simulink model "HLS_VMC_testing"  (R2025a)
settings: Solver=VariableStepAuto  StartTime=0.0  StopTime=0.0001  RelTol=1e-3
InitFcn:
  | fs = 500e6;
values from neighbouring files (symbols this model uses):
  N = length(X)    [outputPlots.m]
undefined symbols (not defined in the file or in its folder): A, es1, i, S, vsva2488, xcvr1602
libraries: hdlBasic x98, hlsBasic x64, aieUtilities x18, dspsrcs4 x15, dspxfrm3 x2, hdlDSPIP x2, hlsUtilities x1, vmcUtilities x1
(part 2 of 4)

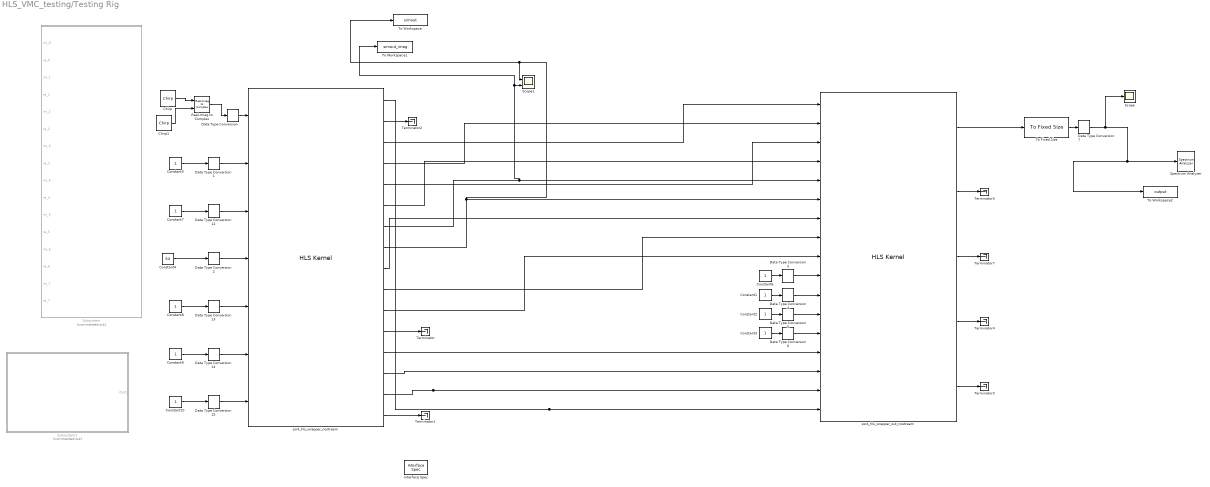
== system HLS_VMC_testing/Testing Rig ==
  Chirp : dspsrcs4/Chirp  sweep=Quadratic  mode=Unidirectional  f0=100e3  f1=100e6  t1=2048/fs  Tsweep=2048/fs  phase=0  Ts=1/fs  spf=1  datatype=double  OutputFrames=off
  Chirp1 : dspsrcs4/Chirp  sweep=Quadratic  mode=Unidirectional  f0=100e3  f1=100e6  t1=2048/fs  Tsweep=2048/fs  phase=pi  Ts=1/fs  spf=1  datatype=double  OutputFrames=off
  Constant{1..3,5..10} (9 alike) : Constant
  Constant4 : Constant  Value=54
  Data Type Conversion : hlsBasic/Data Type Conversion  OutDataType=data type expression  TypeExp='x_sfix64_En63'  Signedness=Signed  WordLength=16  FractionalLength=0  RoundingMode=Truncation to minus infinity  OverflowMode=Wrap around
  Data Type Conversion{1,12..15} (5 alike) : hlsBasic/Data Type Conversion  OutDataType=data type expression  TypeExp='x_ufix1'  Signedness=Signed  WordLength=16  FractionalLength=0  RoundingMode=Truncation to minus infinity  OverflowMode=Wrap around
  Data Type Conversion2 : hlsBasic/Data Type Conversion  OutDataType=data type expression  TypeExp='x_ufix18'  Signedness=Signed  WordLength=16  FractionalLength=0  RoundingMode=Truncation to minus infinity  OverflowMode=Wrap around
  Data Type Conversion{3..6} (4 alike) : hlsBasic/Data Type Conversion  OutDataType=data type expression  TypeExp='x_ufix12'  Signedness=Signed  WordLength=16  FractionalLength=0  RoundingMode=Truncation to minus infinity  OverflowMode=Wrap around
  Data Type Conversion7 : hlsBasic/Data Type Conversion  OutDataType=double  TypeExp=''  Signedness=Signed  WordLength=16  FractionalLength=0  RoundingMode=Truncation to minus infinity  OverflowMode=Wrap around
  Interface Spec : hlsUtilities/Interface Spec  Return=AXI4-Lite Slave@@  InportInterfaces={}  InportHandles={}  InportNames={}  OutportInterfaces={}  OutportHandles={}  OutportNames={}  Mode=AXI4-Lite Slave  InMode1=Default  InVFormat1=N/A  InVComponent1=N/A  InMode2=Default  InVFormat2=N/A  InVComponent2=N/A  InMode3=Default  InVFormat3=N/A  InVComponent3=N/A  InMode4=Default  InVFormat4=N/A  InVComponent4=N/A  InMode5=Default  InVFormat5=N/A  InVComponent5=N/A  InMode6=Default  InVFormat6=N/A  InVComponent6=N/A  InMode7=Default  InVFormat7=N/A  InVComponent7=N/A  InMode8=Default  InVFormat8=N/A  InVComponent8=N/A  OutMode1=Default  OutVFormat1=N/A  OutVComponent1=N/A  OutMode2=Default  OutVFormat2=N/A  OutVComponent2=N/A  OutMode3=Default  OutVFormat3=N/A  OutVComponent3=N/A  OutMode4=Default  OutVFormat4=N/A  OutVComponent4=N/A  OutMode5=Default  OutVFormat5=N/A  OutVComponent5=N/A  OutMode6=Default  OutVFormat6=N/A  OutVComponent6=N/A  OutMode7=Default  OutVFormat7=N/A  OutVComponent7=N/A  OutMode8=Default  OutVFormat8=N/A  OutVComponent8=N/A
  Real-Imag to Complex : hlsBasic/Real-Imag to Complex  Input=Real and imag  ConstantPart=0
  Scope : Scope
      settings: ActiveDisplayYMinimum=-1.249999998402562  ActiveDisplayYMaximum=1.2499999856230579  DataLoggingVariableName=ScopeData5
  Scope1 : Scope  NumInputPorts=2
      settings: ActiveDisplayYMinimum=-1.2499504089355469  ActiveDisplayYMaximum=1.2498588562011719  DataLoggingVariableName=ScopeData6
  Spectrum Analyzer : SpectrumAnalyzer  WindowPosition=[880.000000,470.000000,800.000000,500.000000,]  ScopeFrameLocation=window  WindowInvariantSamplesPerUpdate=on  Span=499999999.99999994  StartFrequency=-249999999.99999997  StopFrequency=249999999.99999997  YLimits=[-36.3231 18.9718]
  Subsystem : Subsystem  Commented=on
  Subsystem1 : Subsystem  Commented=on
  Terminator{,1..5,7} (7 alike) : Terminator
  To Fixed Size : aieUtilities/To Fixed Size  Mode=Stop simulation when input variable-size signal is not full  OutputSize=Inherit: Same as input  CopyMethod=Buffer samples to form output  HasStatusOutput=on
  To Workspace : ToWorkspace  VariableName=simout  SaveFormat=Structure With Time  SampleTime=1/fs
  To Workspace1 : ToWorkspace  VariableName=simout_imag  SaveFormat=Structure With Time  SampleTime=1/fs
  To Workspace2 : ToWorkspace  VariableName=output  SaveFormat=Structure With Time  SampleTime=-1
  ssr4_hls_wrapper_nostream : hlsBasic/HLS Kernel  PortNames={'return'; 'S_AXIS_din_tdata'; 'S_AXIS_din_tready_IN'; 'S_AXIS_din_tvalid_IN'; 'S_AXIS_din_tuser_IN'; 'S_AXIS_din_tlast_IN'; 'S_AXI_aresetn_IN'; 'S_AXI_enable_IN'; 'M_AXIS_dout_tready_OUT'; 'M_AXI_aresetn_OUT'; 'M_AXIS_din_tdata_sample_3_imag'; 'M_AXIS_din_tdata_sample_3_real'; 'M_AXIS_din_tdata_sample_2_imag'; 'M_AXIS_din_tdata_sample_2_real'; 'M_AXIS_din_tdata_sample_1_imag'; 'M_AXIS_din_tdata_sample_1_real'; 'M_AXIS_din_tdata_sample_0_imag'; 'M_AXIS_din_tdata_sample_0_real'; 'M_AXIS_din_tlast_OUT'; 'M_AXIS_din_tuser_scaling'; 'M_AXIS_din_tuser_direction'; 'M_AXIS_din_tuser_point_size'; 'M_AXIS_din_tvalid_OUT'; 'M_AXI_enable_OUT'}  PortSerializedTypes={'{Bv}'; '{R{Tstd::complex{1{t{Tap_fixed{5{t{}64}{t{}1}{t{}5}{t{}3}{t{}0}}}}}}}'; '{R{Tap_uint{1{t{}1}}}}'; '{R{Tap_uint{1{t{}1}}}}'; '{R{Tap_ufixed{5{t{}18}{t{}18}{t{}5}{t{}3}{t{}0}}}}'; '{R{Tap_uint{1{t{}1}}}}'; '{R{Tap_uint{1{t{}1}}}}'; '{R{Tap_uint{1{t{}1}}}}'; '{R{Tap_uint{1{t{}1}}}}'; '{R{Tap_uint{1{t{}1}}}}'; '{R{Tap_fixed{5{t{}16}{t{}1}{t{}0}{t{}3}{t{}0}}}}'; '{R{Tap_fixed{5{t{}16}{t{}1}{t{}0}{t{}3}{t{}0}}}}'; '{R{Tap_fixed{5{t{}16}{t{}1}{t{}0}{t{}3}{t{}0}}}}'; '{R{Tap_fixed{5{t{}16}{t{}1}{t{}0}{t{}3}{t{}0}}}}'; '{R{Tap_fixed{5{t{}16}{t{}1}{t{}0}{t{}3}{t{}0}}}}'; '{R{Tap_fixed{5{t{}16}{t{}1}{t{}0}{t{}3}{t{}0}}}}'; '{R{Tap_fixed{5{t{}16}{t{}1}{t{}0}{t{}3}{t{}0}}}}'; '{R{Tap_fixed{5{t{}16}{t{}1}{t{}0}{t{}3}{t{}0}}}}'; '{R{Tap_uint{1{t{}1}}}}'; '{R{Tap_ufixed{5{t{}13}{t{}1}{t{}5}{t{}3}{t{}0}}}}'; '{R{Tap_uint{1{t{}1}}}}'; '{R{Tap_uint{1{t{}4}}}}'; '{R{Tap_uint{1{t{}1}}}}'; '{R{Tap_uint{1{t{}1}}}}'}  FunctionTemplateSpecKind=none  FunctionTemplateParamNames={}  FunctionTemplateParamKinds={}  FunctionTemplateParamTypes={}  FunctionTemplateParamValues={}  PortSynchronicities={'sync'; 'sync'; 'sync'; 'sync'; 'sync'; 'sync'; 'sync'; 'sync'; 'sync'; 'sync'; 'sync'; 'sync'; 'sync'; 'sync'; 'sync'; 'sync'; 'sync'; 'sync'; 'sync'; 'sync'; 'sync'; 'sync'; 'sync'}  PortSignalSizes={0.000000000000000000e+00; 0.000000000000000000e+00; 0.000000000000000000e+00; 0.000000000000000000e+00; 0.000000000000000000e+00; 0.000000000000000000e+00; 0.000000000000000000e+00; 0.000000000000000000e+00; 0.000000000000000000e+00; 0.000000000000000000e+00; 0.000000000000000000e+00; 0.000000000000000000e+00; 0.000000000000000000e+00; 0.000000000000000000e+00; 0.000000000000000000e+00; 0.000000000000000000e+00; 0.000000000000000000e+00; 0.000000000000000000e+00; 0.000000000000000000e+00; 0.000000000000000000e+00; 0.000000000000000000e+00; 0.000000000000000000e+00; 0.000000000000000000e+00}  PortParameterValues={}  PortAttributesTable={ 'Input', 'S_AXIS_din_tdata', 'std::complex< ap_fixed< 64, 1, 5, 3, 0 > > &', 'sync', ''; 'Input', 'S_AXIS_din_tready_IN', 'ap_uint< 1 > &', 'sync', ''; 'Input', 'S_AXIS_din_tvalid_IN', 'ap_uint< 1 > &', 'sync', ''; 'Input', 'S_AXIS_din_tuser_IN', 'ap_ufixed< 18, 18, 5, 3, 0 > &', 'sync', ''; 'Input', 'S_AXIS_din_tlast_IN', 'ap_uint< 1 > &', 'sync', ''; 'Input', 'S_AXI_aresetn_IN', 'ap_uint< 1 > &', 'sync', ''; 'Input', 'S_AXI_enable_IN', 'ap_uint< 1 > &', 'sync', ''; 'Inout', 'M_AXIS_dout_tready_OUT', 'ap_uint< 1 > &', 'sync', ''; 'Inout', 'M_AXI_aresetn_OUT', 'ap_uint< 1 > &', 'sync', ''; 'Inout', 'M_AXIS_din_tdata_sample_3_imag', 'ap_fixed< 16, 1, 0, 3, 0 > &', 'sync', ''; 'Inout', 'M_AXIS_din_tdata_sample_3_real', 'ap_fixed< 16, 1, 0, 3, 0 > &', 'sync', ''; 'Inout', 'M_AXIS_din_tdata_sample_2_imag', 'ap_fixed< 16, 1, 0, 3, 0 > &', 'sync', ''; 'Inout', 'M_AXIS_din_tdata_sample_2_real', 'ap_fixed< 16, 1, 0, 3, 0 > &', 'sync', ''; 'Inout', 'M_AXIS_din_tdata_sample_1_imag', 'ap_fixed< 16, 1, 0, 3, 0 > &', 'sync', ''; 'Inout', 'M_AXIS_din_tdata_sample_1_real', 'ap_fixed< 16, 1, 0, 3, 0 > &', 'sync', ''; 'Inout', 'M_AXIS_din_tdata_sample_0_imag', 'ap_fixed< 16, 1, 0, 3, 0 > &', 'sync', ''; 'Inout', 'M_AXIS_din_tdata_sample_0_real', 'ap_fixed< 16, 1, 0, 3, 0 > &', 'sync', ''; 'Inout', 'M_AXIS_din_tlast_OUT', 'ap_uint< 1 > &', 'sync', ''; 'Inout', 'M_AXIS_din_tuser_scaling', 'ap_ufixed< 13, 1, 5, 3, 0 > &', 'sync', ''; 'Inout', 'M_AXIS_din_tuser_direction', 'ap_uint< 1 > &', 'sync', ''; 'Inout', 'M_AXIS_din_tuser_point_size', 'ap_uint< 4 > &', 'sync', ''; 'Inout', 'M_AXIS_din_tvalid_OUT', 'ap_uint< 1 > &', 'sync', ''; 'Inout', 'M_AXI_enable_OUT', 'ap_uint< 1 > &', 'sync', '' }  PortAttributesEnablement={'off', 'off', 'off', 'on', 'off';'off', 'off', 'off', 'on', 'off';'off', 'off', 'off', 'on', 'off';'off', 'off', 'off', 'on', 'off';'off', 'off', 'off', 'on', 'off';'off', 'off', 'off', 'on', 'off';'off', 'off', 'off', 'on', 'off';'off', 'off', 'off', 'on', 'off';'off', 'off', 'off', 'on', 'off';'off', 'off', 'off', 'on', 'off';'off', 'off', 'off', 'on', 'off';'off', 'off', 'off', 'on', 'off';'off', 'off', 'off', 'on', 'off';'off', 'off', 'off', 'on', 'off';'off', 'off', 'off', 'on', 'off';'off', 'off', 'off', 'on', 'off';'off', 'off', 'off', 'on', 'off';'off', 'off', 'off', 'on', 'off';'off', 'off', 'off', 'on', 'off';'off', 'off', 'off', 'on', 'off';'off', 'off', 'off', 'on', 'off';'off', 'off', 'off', 'on', 'off';'off', 'off', 'off', 'on', 'off'}  PortParametersTable={}  SampleTime=-1  PortDirectionTable={ 'S_AXIS_din_tdata', 'std::complex< ap_fixed< 64, 1, 5, 3, 0 > > &', 'Input', 'Port'; 'S_AXIS_din_tready_IN', 'ap_uint< 1 > &', 'Input', 'Port'; 'S_AXIS_din_tvalid_IN', 'ap_uint< 1 > &', 'Input', 'Port'; 'S_AXIS_din_tuser_IN', 'ap_ufixed< 18, 18, 5, 3, 0 > &', 'Input', 'Port'; 'S_AXIS_din_tlast_IN', 'ap_uint< 1 > &', 'Input', 'Port'; 'S_AXI_aresetn_IN', 'ap_uint< 1 > &', 'Input', 'Port'; 'S_AXI_enable_IN', 'ap_uint< 1 > &', 'Input', 'Port'; 'M_AXIS_dout_tready_OUT', 'ap_uint< 1 > &', 'Output', 'Port'; 'M_AXI_aresetn_OUT', 'ap_uint< 1 > &', 'Output', 'Port'; 'M_AXIS_din_tdata_sample_3_imag', 'ap_fixed< 16, 1, 0, 3, 0 > &', 'Output', 'Port'; 'M_AXIS_din_tdata_sample_3_real', 'ap_fixed< 16, 1, 0, 3, 0 > &', 'Output', 'Port'; 'M_AXIS_din_tdata_sample_2_imag', 'ap_fixed< 16, 1, 0, 3, 0 > &', 'Output', 'Port'; 'M_AXIS_din_tdata_sample_2_real', 'ap_fixed< 16, 1, 0, 3, 0 > &', 'Output', 'Port'; 'M_AXIS_din_tdata_sample_1_imag', 'ap_fixed< 16, 1, 0, 3, 0 > &', 'Output', 'Port'; 'M_AXIS_din_tdata_sample_1_real', 'ap_fixed< 16, 1, 0, 3, 0 > &', 'Output', 'Port'; 'M_AXIS_din_tdata_sample_0_imag', 'ap_fixed< 16, 1, 0, 3, 0 > &', 'Output', 'Port'; 'M_AXIS_din_tdata_sample_0_real', 'ap_fixed< 16, 1, 0, 3, 0 > &', 'Output', 'Port'; 'M_AXIS_din_tlast_OUT', 'ap_uint< 1 > &', 'Output', 'Port'; 'M_AXIS_din_tuser_scaling', 'ap_ufixed< 13, 1, 5, 3, 0 > &', 'Output', 'Port'; 'M_AXIS_din_tuser_direction', 'ap_uint< 1 > &', 'Output', 'Port'; 'M_AXIS_din_tuser_point_size', 'ap_uint< 4 > &', 'Output', 'Port'; 'M_AXIS_din_tvalid_OUT', 'ap_uint< 1 > &', 'Output', 'Port'; 'M_AXI_enable_OUT', 'ap_uint< 1 > &', 'Output', 'Port' }  FunctionTemplateParams={}  FunctionTemplateParamsEnables={}  FunctionTemplateParamsVisible=off  FunctionDeclTypeOptions=C[1 1]@t7@<empty>  PortDirectionTabVisible=on  ArgDirections={1.000000000000000000e+00; 1.000000000000000000e+00; 1.000000000000000000e+00; 1.000000000000000000e+00; 1.000000000000000000e+00; 1.000000000000000000e+00; 1.000000000000000000e+00; 2.000000000000000000e+00; 2.000000000000000000e+00; 2.000000000000000000e+00; 2.000000000000000000e+00; 2.000000000000000000e+00; 2.000000000000000000e+00; 2.000000000000000000e+00; 2.000000000000000000e+00; 2.000000000000000000e+00; 2.000000000000000000e+00; 2.000000000000000000e+00; 2.000000000000000000e+00; 2.000000000000000000e+00; 2.000000000000000000e+00; 2.000000000000000000e+00; 2.000000000000000000e+00}  ArgInterfaceTypes={1.000000000000000000e+00; 1.000000000000000000e+00; 1.000000000000000000e+00; 1.000000000000000000e+00; 1.000000000000000000e+00; 1.000000000000000000e+00; 1.000000000000000000e+00; 1.000000000000000000e+00; 1.000000000000000000e+00; 1.000000000000000000e+00; 1.000000000000000000e+00; 1.000000000000000000e+00; 1.000000000000000000e+00; 1.000000000000000000e+00; 1.000000000000000000e+00; 1.000000000000000000e+00; 1.000000000000000000e+00; 1.000000000000000000e+00; 1.000000000000000000e+00; 1.000000000000000000e+00; 1.000000000000000000e+00; 1.000000000000000000e+00; 1.000000000000000000e+00}  FunctionIndex=1  FormalArgDecls={'std::complex< ap_fixed< 64, 1, 5, 3, 0 > > & S_AXIS_din_tdata', 'ap_uint< 1 > & S_AXIS_din_tready_IN', 'ap_uint< 1 > & S_AXIS_din_tvalid_IN', 'ap_ufixed< 18, 18, 5, 3, 0 > & S_AXIS_din_tuser_IN', 'ap_uint< 1 > & S_AXIS_din_tlast_IN', 'ap_uint< 1 > & S_AXI_aresetn_IN', 'ap_uint< 1 > & S_AXI_enable_IN', 'ap_uint< 1 > & M_AXIS_dout_tready_OUT', 'ap_uint< 1 > & M_AXI_aresetn_OUT', 'ap_fixed< 16, 1, 0, 3, 0 > & M_AXIS_din_tdata_sample_3_imag', 'ap_fixed< 16, 1, 0, 3, 0 > & M_AXIS_din_tdata_sample_3_real', 'ap_fixed< 16, 1, 0, 3, 0 > & M_AXIS_din_tdata_sample_2_imag', 'ap_fixed< 16, 1, 0, 3, 0 > & M_AXIS_din_tdata_sample_2_real', 'ap_fixed< 16, 1, 0, 3, 0 > & M_AXIS_din_tdata_sample_1_imag', 'ap_fixed< 16, 1, 0, 3, 0 > & M_AXIS_din_tdata_sample_1_real', 'ap_fixed< 16, 1, 0, 3, 0 > & M_AXIS_din_tdata_sample_0_imag', 'ap_fixed< 16, 1, 0, 3, 0 > & M_AXIS_din_tdata_sample_0_real', 'ap_uint< 1 > & M_AXIS_din_tlast_OUT', 'ap_ufixed< 13, 1, 5, 3, 0 > & M_AXIS_din_tuser_scaling', 'ap_uint< 1 > & M_AXIS_din_tuser_direction', 'ap_uint< 4 > & M_AXIS_din_tuser_point_size', 'ap_uint< 1 > & M_AXIS_din_tvalid_OUT', 'ap_uint< 1 > & M_AXI_enable_OUT'}  SimLibPath=''  FunctionTabVisible=on  FunctionDescription=void ssr4_hls_wrapper_nostream(std::complex< ap_fixed< 64, 1, 5, 3, 0 > > & S_AXIS_din_tdata, ap_uint< 1 > & S_AXIS_din_tready_IN, ap_uint< 1 > & S_AXIS_din_tvalid_IN, ap_ufixed< 18, 18, 5, 3, 0 > & S_AXIS_din_tuser_IN, ap_uint< 1 > & S_AXIS_din_tlast_IN, ap_uint< 1 > & S_AXI_aresetn_IN, ap_uint< 1 > & S_AXI_enable_IN, ap_uint< 1 > & M_AXIS_dout_tready_OUT, ap_uint< 1 > & M_AXI_aresetn_OUT, ap_fixed< 16, 1, 0, 3, 0 > & M_AXIS_din_tdata_sample_3_imag, ap_fixed< 16, 1, 0, 3, 0 > & M_AXIS_din_tdata_sample_3_real, ap_fixed< 16, 1, 0, 3, 0 > & M_AXIS_din_tdata_sample_2_imag, ap_fixed< 16, 1, 0, 3, 0 > & M_AXIS_din_tdata_sample_2_real, ap_fixed< 16, 1, 0, 3, 0 > & M_AXIS_din_tdata_sample_1_imag, ap_fixed< 16, 1, 0, 3, 0 > & M_AXIS_din_tdata_sample_1_real, ap_fixed< 16, 1, 0, 3, 0 > & M_AXIS_din_tdata_sample_0_imag, ap_fixed< 16, 1, 0, 3, 0 > & M_AXIS_din_tdata_sample_0_real, ap_uint< 1 > & M_AXIS_din_tlast_OUT, ap_ufixed< 13, 1, 5, 3, 0 > & M_AXIS_din_tuser_scaling, ap_uint< 1 > & M_AXIS_din_tuser_direction, ap_uint< 4 > & M_AXIS_din_tuser_point_size, ap_uint< 1 > & M_AXIS_din_tvalid_OUT, ap_uint< 1 > & M_AXI_enable_OUT)  blockJsonConstraints=[]  deprecateConstraints=0  KernelHeaderFile=src/wrapperin.h  KernelFunction=ssr4_hls_wrapper_nostream  KernelFunctionSelect=<empty>  KernelSourceFile=src/wrapperin.cpp  KernelSearchPaths={}  PreProcOptions={}
  ssr4_hls_wrapper_out_nostream : hlsBasic/HLS Kernel  PortNames={'return'; 'S_AXIS_din_tdata_sample_3_imag'; 'S_AXIS_din_tdata_sample_3_real'; 'S_AXIS_din_tdata_sample_2_imag'; 'S_AXIS_din_tdata_sample_2_real'; 'S_AXIS_din_tdata_sample_1_imag'; 'S_AXIS_din_tdata_sample_1_real'; 'S_AXIS_din_tdata_sample_0_imag'; 'S_AXIS_din_tdata_sample_0_real'; 'S_AXIS_din_tlast_IN'; 'S_AXIS_din_tuser_index_3'; 'S_AXIS_din_tuser_index_2'; 'S_AXIS_din_tuser_index_1'; 'S_AXIS_din_tuser_index_0'; 'S_AXIS_din_tuser_direction'; 'S_AXIS_din_tuser_point_size'; 'S_AXIS_tvalid_IN'; 'S_AXIS_dout_tready_OUT'; 'M_AXIS_dout_tdata'; 'M_AXIS_dout_tlast_OUT'; 'M_AXIS_dout_tready_OUT'; 'M_AXIS_dout_tuser_OUT'; 'M_AXIS_dout_tvalid_OUT'}  PortSerializedTypes={'{Bv}'; '{R{Tap_fixed{5{t{}16}{t{}1}{t{}0}{t{}3}{t{}0}}}}'; '{R{Tap_fixed{5{t{}16}{t{}1}{t{}0}{t{}3}{t{}0}}}}'; '{R{Tap_fixed{5{t{}16}{t{}1}{t{}0}{t{}3}{t{}0}}}}'; '{R{Tap_fixed{5{t{}16}{t{}1}{t{}0}{t{}3}{t{}0}}}}'; '{R{Tap_fixed{5{t{}16}{t{}1}{t{}0}{t{}3}{t{}0}}}}'; '{R{Tap_fixed{5{t{}16}{t{}1}{t{}0}{t{}3}{t{}0}}}}'; '{R{Tap_fixed{5{t{}16}{t{}1}{t{}0}{t{}3}{t{}0}}}}'; '{R{Tap_fixed{5{t{}16}{t{}1}{t{}0}{t{}3}{t{}0}}}}'; '{R{Tap_uint{1{t{}1}}}}'; '{R{Tap_uint{1{t{}12}}}}'; '{R{Tap_uint{1{t{}12}}}}'; '{R{Tap_uint{1{t{}12}}}}'; '{R{Tap_uint{1{t{}12}}}}'; '{R{Tap_uint{1{t{}1}}}}'; '{R{Tap_uint{1{t{}4}}}}'; '{R{Tap_uint{1{t{}1}}}}'; '{R{Tap_uint{1{t{}1}}}}'; '{R{Tstd::complex{1{t{Tap_fixed{5{t{}64}{t{}1}{t{}0}{t{}3}{t{}0}}}}}}}'; '{R{Tap_uint{1{t{}1}}}}'; '{R{Tap_uint{1{t{}1}}}}'; '{R{Tap_uint{1{t{}53}}}}'; '{R{Tap_uint{1{t{}1}}}}'}  FunctionTemplateSpecKind=none  FunctionTemplateParamNames={}  FunctionTemplateParamKinds={}  FunctionTemplateParamTypes={}  FunctionTemplateParamValues={}  PortSynchronicities={'sync'; 'sync'; 'sync'; 'sync'; 'sync'; 'sync'; 'sync'; 'sync'; 'sync'; 'sync'; 'sync'; 'sync'; 'sync'; 'sync'; 'sync'; 'sync'; 'sync'; 'sync'; 'sync'; 'sync'; 'sync'; 'sync'}  PortSignalSizes={0.000000000000000000e+00; 0.000000000000000000e+00; 0.000000000000000000e+00; 0.000000000000000000e+00; 0.000000000000000000e+00; 0.000000000000000000e+00; 0.000000000000000000e+00; 0.000000000000000000e+00; 0.000000000000000000e+00; 0.000000000000000000e+00; 0.000000000000000000e+00; 0.000000000000000000e+00; 0.000000000000000000e+00; 0.000000000000000000e+00; 0.000000000000000000e+00; 0.000000000000000000e+00; 0.000000000000000000e+00; 0.000000000000000000e+00; 0.000000000000000000e+00; 0.000000000000000000e+00; 0.000000000000000000e+00; 0.000000000000000000e+00}  PortParameterValues={}  PortAttributesTable={ 'Input', 'S_AXIS_din_tdata_sample_3_imag', 'ap_fixed< 16, 1, 0, 3, 0 > &', 'sync', ''; 'Input', 'S_AXIS_din_tdata_sample_3_real', 'ap_fixed< 16, 1, 0, 3, 0 > &', 'sync', ''; 'Input', 'S_AXIS_din_tdata_sample_2_imag', 'ap_fixed< 16, 1, 0, 3, 0 > &', 'sync', ''; 'Input', 'S_AXIS_din_tdata_sample_2_real', 'ap_fixed< 16, 1, 0, 3, 0 > &', 'sync', ''; 'Input', 'S_AXIS_din_tdata_sample_1_imag', 'ap_fixed< 16, 1, 0, 3, 0 > &', 'sync', ''; 'Input', 'S_AXIS_din_tdata_sample_1_real', 'ap_fixed< 16, 1, 0, 3, 0 > &', 'sync', ''; 'Input', 'S_AXIS_din_tdata_sample_0_imag', 'ap_fixed< 16, 1, 0, 3, 0 > &', 'sync', ''; 'Input', 'S_AXIS_din_tdata_sample_0_real', 'ap_fixed< 16, 1, 0, 3, 0 > &', 'sync', ''; 'Input', 'S_AXIS_din_tlast_IN', 'ap_uint< 1 > &', 'sync', ''; 'Input', 'S_AXIS_din_tuser_index_3', 'ap_uint< 12 > &', 'sync', ''; 'Input', 'S_AXIS_din_tuser_index_2', 'ap_uint< 12 > &', 'sync', ''; 'Input', 'S_AXIS_din_tuser_index_1', 'ap_uint< 12 > &', 'sync', ''; 'Input', 'S_AXIS_din_tuser_index_0', 'ap_uint< 12 > &', 'sync', ''; 'Input', 'S_AXIS_din_tuser_direction', 'ap_uint< 1 > &', 'sync', ''; 'Input', 'S_AXIS_din_tuser_point_size', 'ap_uint< 4 > &', 'sync', ''; 'Input', 'S_AXIS_tvalid_IN', 'ap_uint< 1 > &', 'sync', ''; 'Input', 'S_AXIS_dout_tready_OUT', 'ap_uint< 1 > &', 'sync', ''; 'Inout', 'M_AXIS_dout_tdata', 'std::complex< ap_fixed< 64, 1, 0, 3, 0 > > &', 'sync', ''; 'Inout', 'M_AXIS_dout_tlast_OUT', 'ap_uint< 1 > &', 'sync', ''; 'Inout', 'M_AXIS_dout_tready_OUT', 'ap_uint< 1 > &', 'sync', ''; 'Inout', 'M_AXIS_dout_tuser_OUT', 'ap_uint< 53 > &', 'sync', ''; 'Inout', 'M_AXIS_dout_tvalid_OUT', 'ap_uint< 1 > &', 'sync', '' }  PortAttributesEnablement={'off', 'off', 'off', 'on', 'off';'off', 'off', 'off', 'on', 'off';'off', 'off', 'off', 'on', 'off';'off', 'off', 'off', 'on', 'off';'off', 'off', 'off', 'on', 'off';'off', 'off', 'off', 'on', 'off';'off', 'off', 'off', 'on', 'off';'off', 'off', 'off', 'on', 'off';'off', 'off', 'off', 'on', 'off';'off', 'off', 'off', 'on', 'off';'off', 'off', 'off', 'on', 'off';'off', 'off', 'off', 'on', 'off';'off', 'off', 'off', 'on', 'off';'off', 'off', 'off', 'on', 'off';'off', 'off', 'off', 'on', 'off';'off', 'off', 'off', 'on', 'off';'off', 'off', 'off', 'on', 'off';'off', 'off', 'off', 'on', 'off';'off', 'off', 'off', 'on', 'off';'off', 'off', 'off', 'on', 'off';'off', 'off', 'off', 'on', 'off';'off', 'off', 'off', 'on', 'off'}  PortParametersTable={}  SampleTime=-1  PortDirectionTable={ 'S_AXIS_din_tdata_sample_3_imag', 'ap_fixed< 16, 1, 0, 3, 0 > &', 'Input', 'Port'; 'S_AXIS_din_tdata_sample_3_real', 'ap_fixed< 16, 1, 0, 3, 0 > &', 'Input', 'Port'; 'S_AXIS_din_tdata_sample_2_imag', 'ap_fixed< 16, 1, 0, 3, 0 > &', 'Input', 'Port'; 'S_AXIS_din_tdata_sample_2_real', 'ap_fixed< 16, 1, 0, 3, 0 > &', 'Input', 'Port'; 'S_AXIS_din_tdata_sample_1_imag', 'ap_fixed< 16, 1, 0, 3, 0 > &', 'Input', 'Port'; 'S_AXIS_din_tdata_sample_1_real', 'ap_fixed< 16, 1, 0, 3, 0 > &', 'Input', 'Port'; 'S_AXIS_din_tdata_sample_0_imag', 'ap_fixed< 16, 1, 0, 3, 0 > &', 'Input', 'Port'; 'S_AXIS_din_tdata_sample_0_real', 'ap_fixed< 16, 1, 0, 3, 0 > &', 'Input', 'Port'; 'S_AXIS_din_tlast_IN', 'ap_uint< 1 > &', 'Input', 'Port'; 'S_AXIS_din_tuser_index_3', 'ap_uint< 12 > &', 'Input', 'Port'; 'S_AXIS_din_tuser_index_2', 'ap_uint< 12 > &', 'Input', 'Port'; 'S_AXIS_din_tuser_index_1', 'ap_uint< 12 > &', 'Input', 'Port'; 'S_AXIS_din_tuser_index_0', 'ap_uint< 12 > &', 'Input', 'Port'; 'S_AXIS_din_tuser_direction', 'ap_uint< 1 > &', 'Input', 'Port'; 'S_AXIS_din_tuser_point_size', 'ap_uint< 4 > &', 'Input', 'Port'; 'S_AXIS_tvalid_IN', 'ap_uint< 1 > &', 'Input', 'Port'; 'S_AXIS_dout_tready_OUT', 'ap_uint< 1 > &', 'Input', 'Port'; 'M_AXIS_dout_tdata', 'std::complex< ap_fixed< 64, 1, 0, 3, 0 > > &', 'Output', 'Port'; 'M_AXIS_dout_tlast_OUT', 'ap_uint< 1 > &', 'Output', 'Port'; 'M_AXIS_dout_tready_OUT', 'ap_uint< 1 > &', 'Output', 'Port'; 'M_AXIS_dout_tuser_OUT', 'ap_uint< 53 > &', 'Output', 'Port'; 'M_AXIS_dout_tvalid_OUT', 'ap_uint< 1 > &', 'Output', 'Port' }  FunctionTemplateParams={}  FunctionTemplateParamsEnables={}  FunctionTemplateParamsVisible=off  FunctionDeclTypeOptions=C[1 1]@t7@<empty>  PortDirectionTabVisible=on  ArgDirections={1.000000000000000000e+00; 1.000000000000000000e+00; 1.000000000000000000e+00; 1.000000000000000000e+00; 1.000000000000000000e+00; 1.000000000000000000e+00; 1.000000000000000000e+00; 1.000000000000000000e+00; 1.000000000000000000e+00; 1.000000000000000000e+00; 1.000000000000000000e+00; 1.000000000000000000e+00; 1.000000000000000000e+00; 1.000000000000000000e+00; 1.000000000000000000e+00; 1.000000000000000000e+00; 1.000000000000000000e+00; 2.000000000000000000e+00; 2.000000000000000000e+00; 2.000000000000000000e+00; 2.000000000000000000e+00; 2.000000000000000000e+00}  ArgInterfaceTypes={1.000000000000000000e+00; 1.000000000000000000e+00; 1.000000000000000000e+00; 1.000000000000000000e+00; 1.000000000000000000e+00; 1.000000000000000000e+00; 1.000000000000000000e+00; 1.000000000000000000e+00; 1.000000000000000000e+00; 1.000000000000000000e+00; 1.000000000000000000e+00; 1.000000000000000000e+00; 1.000000000000000000e+00; 1.000000000000000000e+00; 1.000000000000000000e+00; 1.000000000000000000e+00; 1.000000000000000000e+00; 1.000000000000000000e+00; 1.000000000000000000e+00; 1.000000000000000000e+00; 1.000000000000000000e+00; 1.000000000000000000e+00}  FunctionIndex=1  FormalArgDecls={'ap_fixed< 16, 1, 0, 3, 0 > & S_AXIS_din_tdata_sample_3_imag', 'ap_fixed< 16, 1, 0, 3, 0 > & S_AXIS_din_tdata_sample_3_real', 'ap_fixed< 16, 1, 0, 3, 0 > & S_AXIS_din_tdata_sample_2_imag', 'ap_fixed< 16, 1, 0, 3, 0 > & S_AXIS_din_tdata_sample_2_real', 'ap_fixed< 16, 1, 0, 3, 0 > & S_AXIS_din_tdata_sample_1_imag', 'ap_fixed< 16, 1, 0, 3, 0 > & S_AXIS_din_tdata_sample_1_real', 'ap_fixed< 16, 1, 0, 3, 0 > & S_AXIS_din_tdata_sample_0_imag', 'ap_fixed< 16, 1, 0, 3, 0 > & S_AXIS_din_tdata_sample_0_real', 'ap_uint< 1 > & S_AXIS_din_tlast_IN', 'ap_uint< 12 > & S_AXIS_din_tuser_index_3', 'ap_uint< 12 > & S_AXIS_din_tuser_index_2', 'ap_uint< 12 > & S_AXIS_din_tuser_index_1', 'ap_uint< 12 > & S_AXIS_din_tuser_index_0', 'ap_uint< 1 > & S_AXIS_din_tuser_direction', 'ap_uint< 4 > & S_AXIS_din_tuser_point_size', 'ap_uint< 1 > & S_AXIS_tvalid_IN', 'ap_uint< 1 > & S_AXIS_dout_tready_OUT', 'std::complex< ap_fixed< 64, 1, 0, 3, 0 > > & M_AXIS_dout_tdata', 'ap_uint< 1 > & M_AXIS_dout_tlast_OUT', 'ap_uint< 1 > & M_AXIS_dout_tready_OUT', 'ap_uint< 53 > & M_AXIS_dout_tuser_OUT', 'ap_uint< 1 > & M_AXIS_dout_tvalid_OUT'}  SimLibPath=''  FunctionTabVisible=on  FunctionDescription=void ssr4_hls_wrapper_out_nostream(ap_fixed< 16, 1, 0, 3, 0 > & S_AXIS_din_tdata_sample_3_imag, ap_fixed< 16, 1, 0, 3, 0 > & S_AXIS_din_tdata_sample_3_real, ap_fixed< 16, 1, 0, 3, 0 > & S_AXIS_din_tdata_sample_2_imag, ap_fixed< 16, 1, 0, 3, 0 > & S_AXIS_din_tdata_sample_2_real, ap_fixed< 16, 1, 0, 3, 0 > & S_AXIS_din_tdata_sample_1_imag, ap_fixed< 16, 1, 0, 3, 0 > & S_AXIS_din_tdata_sample_1_real, ap_fixed< 16, 1, 0, 3, 0 > & S_AXIS_din_tdata_sample_0_imag, ap_fixed< 16, 1, 0, 3, 0 > & S_AXIS_din_tdata_sample_0_real, ap_uint< 1 > & S_AXIS_din_tlast_IN, ap_uint< 12 > & S_AXIS_din_tuser_index_3, ap_uint< 12 > & S_AXIS_din_tuser_index_2, ap_uint< 12 > & S_AXIS_din_tuser_index_1, ap_uint< 12 > & S_AXIS_din_tuser_index_0, ap_uint< 1 > & S_AXIS_din_tuser_direction, ap_uint< 4 > & S_AXIS_din_tuser_point_size, ap_uint< 1 > & S_AXIS_tvalid_IN, ap_uint< 1 > & S_AXIS_dout_tready_OUT, std::complex< ap_fixed< 64, 1, 0, 3, 0 > > & M_AXIS_dout_tdata, ap_uint< 1 > & M_AXIS_dout_tlast_OUT, ap_uint< 1 > & M_AXIS_dout_tready_OUT, ap_uint< 53 > & M_AXIS_dout_tuser_OUT, ap_uint< 1 > & M_AXIS_dout_tvalid_OUT)  blockJsonConstraints=[]  deprecateConstraints=0  KernelHeaderFile=wrapper_out_src/wrapperout.h  KernelFunction=ssr4_hls_wrapper_out_nostream  KernelFunctionSelect=<empty>  KernelSourceFile=wrapper_out_src/wrapperout.cpp  KernelSearchPaths={}  PreProcOptions={}
  wires:
  ssr4_hls_wrapper_nostream/7 -> ssr4_hls_wrapper_out_nostream/5, To Workspace1/1, Scope1/2
  ssr4_hls_wrapper_nostream/11 -> ssr4_hls_wrapper_out_nostream/9
  ssr4_hls_wrapper_nostream/12 -> Terminator/1
  ssr4_hls_wrapper_nostream/13 -> ssr4_hls_wrapper_out_nostream/14
  ssr4_hls_wrapper_nostream/14 -> ssr4_hls_wrapper_out_nostream/15
  ssr4_hls_wrapper_nostream/15 -> ssr4_hls_wrapper_out_nostream/16
  ssr4_hls_wrapper_nostream/16 -> Terminator1/1
  ssr4_hls_wrapper_nostream/2 -> Terminator2/1
  Data Type Conversion2/1 -> ssr4_hls_wrapper_nostream/4
  Data Type Conversion1/1 -> ssr4_hls_wrapper_nostream/2
  Real-Imag to Complex/1 -> Data Type Conversion/1
  Constant4/1 -> Data Type Conversion2/1
  Constant5/1 -> Data Type Conversion1/1
  Data Type Conversion3/1 -> ssr4_hls_wrapper_out_nostream/10
  Constant6/1 -> Data Type Conversion3/1
  Data Type Conversion4/1 -> ssr4_hls_wrapper_out_nostream/11
  Constant1/1 -> Data Type Conversion4/1
  Data Type Conversion5/1 -> ssr4_hls_wrapper_out_nostream/12
  Constant2/1 -> Data Type Conversion5/1
  Data Type Conversion6/1 -> ssr4_hls_wrapper_out_nostream/13
  Constant3/1 -> Data Type Conversion6/1
  ssr4_hls_wrapper_nostream/8 -> ssr4_hls_wrapper_out_nostream/6, To Workspace/1, Scope1/1
  Chirp/1 -> Real-Imag to Complex/1
  Chirp1/1 -> Real-Imag to Complex/2
  Data Type Conversion/1 -> ssr4_hls_wrapper_nostream/1
  To Fixed Size/1 -> Data Type Conversion7/1
  Data Type Conversion7/1 -> Scope/1, To Workspace2/1, Spectrum Analyzer/1
  ssr4_hls_wrapper_nostream/1 -> ssr4_hls_wrapper_out_nostream/17
  Data Type Conversion12/1 -> ssr4_hls_wrapper_nostream/3
  Constant7/1 -> Data Type Conversion12/1
  Data Type Conversion13/1 -> ssr4_hls_wrapper_nostream/5
  Constant8/1 -> Data Type Conversion13/1
  Data Type Conversion14/1 -> ssr4_hls_wrapper_nostream/6
  Constant9/1 -> Data Type Conversion14/1
  Data Type Conversion15/1 -> ssr4_hls_wrapper_nostream/7
  Constant10/1 -> Data Type Conversion15/1
  ssr4_hls_wrapper_nostream/3 -> ssr4_hls_wrapper_out_nostream/1
  ssr4_hls_wrapper_nostream/4 -> ssr4_hls_wrapper_out_nostream/2
  ssr4_hls_wrapper_nostream/5 -> ssr4_hls_wrapper_out_nostream/3
  ssr4_hls_wrapper_nostream/6 -> ssr4_hls_wrapper_out_nostream/4
  ssr4_hls_wrapper_nostream/9 -> ssr4_hls_wrapper_out_nostream/7
  ssr4_hls_wrapper_nostream/10 -> ssr4_hls_wrapper_out_nostream/8
  ssr4_hls_wrapper_out_nostream/5 -> Terminator3/1
  ssr4_hls_wrapper_out_nostream/4 -> Terminator4/1
  ssr4_hls_wrapper_out_nostream/2 -> Terminator5/1
  ssr4_hls_wrapper_out_nostream/3 -> Terminator7/1
  ssr4_hls_wrapper_out_nostream/1 -> To Fixed Size/1

== system HLS_VMC_testing/Versal FFT HLS Wrapper ==
  S_AXIS_din_tdata : Inport
  " Scaling" : hdlBasic/Gateway In  gui_display_data_type=Fixed-point  arith_type=Unsigned  n_bits=13  bin_pt=13  preci_type=Single  exp_width=8  frac_width=24  rows=1  columns=1  quantization="Round  (unbiased: +/- Inf)"  overflow=Saturate  period=1/fs  UseAsADC=off  ADCChannel='1'  interface=None  automatic_assignment=on  address_offset=hex2dec('00')  intf_name=''  intf_description=''  default_value=0  timing_constraint=None  locs_specified=off  LOCs={}  io_standard={}  inherit_from_input=off  hdl_port=on  XmcBlockStatus=1  maskContainerNames=group4  block_type=gatewayin  block_config=sysgen:gateway_in_config  block_width_w=590  block_height_w=620  block_width=640  block_height=850
  Concat : hdlBasic/Concat  num_inputs=3  XmcBlockStatus=1  maskContainerNames=group1  block_type=concat  block_config=sysgen:Concat_config
  Direction : hdlBasic/Gateway In  gui_display_data_type=Boolean  arith_type=Boolean  n_bits=16  bin_pt=14  preci_type=Single  exp_width=8  frac_width=24  rows=1  columns=1  quantization="Round  (unbiased: +/- Inf)"  overflow=Saturate  period=1/fs  UseAsADC=off  ADCChannel='1'  interface=None  automatic_assignment=on  address_offset=hex2dec('00')  intf_name=''  intf_description=''  default_value=0  timing_constraint=None  locs_specified=off  LOCs={}  io_standard={}  inherit_from_input=off  hdl_port=on  XmcBlockStatus=1  maskContainerNames=group4  block_type=gatewayin  block_config=sysgen:gateway_in_config  block_width_w=590  block_height_w=620  block_width=640  block_height=850
  Display1 : Display
  Point Size : hdlBasic/Gateway In  gui_display_data_type=Fixed-point  arith_type=Unsigned  n_bits=4  bin_pt=0  preci_type=Single  exp_width=8  frac_width=24  rows=1  columns=1  quantization="Round  (unbiased: +/- Inf)"  overflow=Saturate  period=1/fs  UseAsADC=off  ADCChannel='1'  interface=None  automatic_assignment=on  address_offset=hex2dec('00')  intf_name=''  intf_description=''  default_value=0  timing_constraint=None  locs_specified=off  LOCs={}  io_standard={}  inherit_from_input=off  hdl_port=on  XmcBlockStatus=1  maskContainerNames=group4  block_type=gatewayin  block_config=sysgen:gateway_in_config  block_width_w=590  block_height_w=620  block_width=640  block_height=850
  Scope : Scope
      settings: ActiveDisplayYMinimum=-0.12499999999999997  ActiveDisplayYMaximum=1.125  DataLoggingVariableName=ScopeData3
  Shift : hdlBasic/Shift  shift_dir=Left  shift_bits=13  en=off  latency=0  precision=User Defined  arith_type=Unsigned  n_bits=13  bin_pt=0  quantization=Truncate  overflow=Wrap  XmcBlockStatus=1  maskContainerNames=group2  block_type=shift  block_config=sysgen:Shift_config
  TLAST_DELAY : DiscretePulseGenerator  Period=FFT_SIZE  PhaseDelay=FFT_SIZE - 1  SampleTime=1/fs
  TUSER_Direction : Constant  Value=tuser_dir  SampleTime=1/fs
  TUSER_PointSIze : Constant  Value=tuser_ps  SampleTime=1/fs
  TUSER_Scaling : Constant  Value=tuser  SampleTime=1/fs
  mask_level_wrapper : Subsystem
  M_AXIS_dout_tdata : Outport
  dout_tvalid : Outport  Port=2
  wires:
  mask_level_wrapper/1(M_AXIS_dout_tdata) -> M_AXIS_dout_tdata/1
  S_AXIS_din_tdata/1 -> mask_level_wrapper/1(S_AXIS_din_tdata)
  TUSER_Direction/1 -> Direction/1
  TUSER_PointSIze/1 -> Point Size/1
  TUSER_Scaling/1 -> " Scaling"/1
  Point Size/1 -> Concat/3
  Direction/1 -> Concat/2
  mask_level_wrapper/2(dout_tvalid) -> dout_tvalid/1
  Concat/1 -> mask_level_wrapper/2(S_AXIS_din_tuser)
  TLAST_DELAY/1 -> mask_level_wrapper/3(S_AXIS_din_tlast)
  " Scaling"/1 -> Shift/1
  Shift/1 -> Concat/1

== system HLS_VMC_testing/Versal FFT HLS Wrapper1 ==
  S_AXIS_din_tdata : Inport
  Constant : Constant  Value=tuser
  Constant1 : Constant  Value=tuser_dir
  Constant2 : Constant  Value=tuser_ps
  Data Type Conversion : hlsBasic/Data Type Conversion  OutDataType=double  TypeExp=''  Signedness=Signed  WordLength=16  FractionalLength=0  RoundingMode=Truncation to minus infinity  OverflowMode=Wrap around
  TLAST_DELAY : DiscretePulseGenerator  Period=FFT_SIZE  PhaseDelay=FFT_SIZE - 1  SampleTime=1/fs
  TUSER formatting : Subsystem
  mask_level_wrapper : Subsystem
  M_AXIS_dout_tdata : Outport
  M_AXIS_dout_tvalid : Outport  Port=2
  wires:
  mask_level_wrapper/1(M_AXIS_dout_tdata_) -> M_AXIS_dout_tdata/1
  S_AXIS_din_tdata/1 -> mask_level_wrapper/1(S_AXIS_din_tdata_)
  TLAST_DELAY/1 -> mask_level_wrapper/3(S_AXIS_din_tlast_)
  mask_level_wrapper/2(tvalid) -> M_AXIS_dout_tvalid/1
  TUSER formatting/1(S_AXIS_din_tuser_) -> Data Type Conversion/1
  Constant/1 -> TUSER formatting/1(In1)
  Constant1/1 -> TUSER formatting/2(In2)
  Constant2/1 -> TUSER formatting/3(In3)
  Data Type Conversion/1 -> mask_level_wrapper/2(S_AXIS_din_tuser_)

== system HLS_VMC_testing/Input Stimuli1/Pre Processing ==
  In1 : Inport
  Buffer2 : Buffer  N=1  OutputFrames=off
  Complex to Real-Imag : ComplexToRealImag
  Matrix Concatenate1 : Concatenate  Mode=Multidimensional array
  Reshape1 : Reshape  OutputDimensionality=Customize  OutputDimensions=[1, 2]
  Reshape2 : Reshape  OutputDimensions=[1, 10]
  Transpose : Math  Operator=transpose
  HDL_FFT : Outport
  wires:
  Transpose/1 -> Reshape2/1
  Buffer2/1 -> HDL_FFT/1  "HDL_FFT"
  Reshape2/1 -> Buffer2/1  "HDL_FFT"
  Matrix Concatenate1/1 -> Reshape1/1
  Reshape1/1 -> Transpose/1
  In1/1 -> Complex to Real-Imag/1
  Complex to Real-Imag/1 -> Matrix Concatenate1/1
  Complex to Real-Imag/2 -> Matrix Concatenate1/2

== system HLS_VMC_testing/Output Plotting/Subsystem ==
  In1 : Inport
  Enable : EnablePort
  Abs : Abs  SaturateOnIntegerOverflow=off
  Buffer : Buffer  N=1024  OutputFrames=off
  Out1 : Outport
  wires:
  In1/1 -> Abs/1
  Buffer/1 -> Out1/1
  Abs/1 -> Buffer/1

== system HLS_VMC_testing/Output Plotting1/Subsystem ==
  In1 : Inport
  Abs : Abs  SaturateOnIntegerOverflow=off
  Buffer : Buffer  N=1024  OutputFrames=off
  Out1 : Outport
  wires:
  In1/1 -> Abs/1
  Buffer/1 -> Out1/1
  Abs/1 -> Buffer/1

== system HLS_VMC_testing/Subsystem/Subsystem ==
  In1 : Inport
  In2 : Inport  Port=2
  Buffer2 : Buffer  N=1  OutputFrames=off
  Complex to Real-Imag : ComplexToRealImag  Commented=on
  Matrix Concatenate1 : Concatenate  Mode=Multidimensional array
  Reshape1 : Reshape  OutputDimensionality=Customize  OutputDimensions=[1, 2]
  Reshape2 : Reshape  OutputDimensions=[1, 10]
  Transpose : Math  Operator=transpose
  HDL_FFT : Outport
  wires:
  Transpose/1 -> Reshape2/1
  Buffer2/1 -> HDL_FFT/1  "HDL_FFT"
  Reshape2/1 -> Buffer2/1  "HDL_FFT"
  Matrix Concatenate1/1 -> Reshape1/1
  Reshape1/1 -> Transpose/1
  In1/1 -> Matrix Concatenate1/1
  In2/1 -> Matrix Concatenate1/2

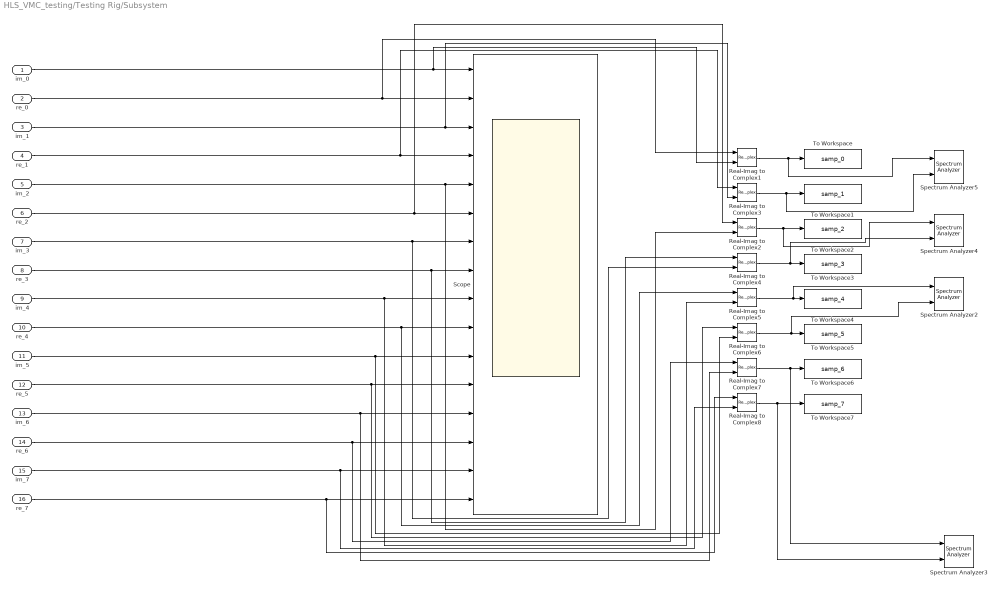
== system HLS_VMC_testing/Testing Rig/Subsystem ==
  im_0 : Inport
  re_0 : Inport  Port=2
  im_1 : Inport  Port=3
  re_1 : Inport  Port=4
  im_2 : Inport  Port=5
  re_2 : Inport  Port=6
  im_3 : Inport  Port=7
  re_3 : Inport  Port=8
  im_4 : Inport  Port=9
  re_4 : Inport  Port=10
  im_5 : Inport  Port=11
  re_5 : Inport  Port=12
  im_6 : Inport  Port=13
  re_6 : Inport  Port=14
  im_7 : Inport  Port=15
  re_7 : Inport  Port=16
  Real-Imag to Complex{1..8} (8 alike) : RealImagToComplex
  Scope : Scope  NumInputPorts=16
      settings: ActiveDisplayYMinimum=-1.25  ActiveDisplayYMaximum=1.25
  Spectrum Analyzer{2..5} (4 alike) : SpectrumAnalyzer  NumInputPorts=2  WindowPosition=[1.000000,1.000000,1920.000000,1029.000000,]  ScopeFrameLocation=window  ViewType=Spectrum and spectrogram  WindowInvariantSamplesPerUpdate=on  YLimits=[-3603.4449 -2802.6794]  ColorLimits=[-3603.4449 -2802.6794]
  To Workspace : ToWorkspace  VariableName=samp_0  SaveFormat=Structure With Time  SampleTime=-1
  To Workspace1 : ToWorkspace  VariableName=samp_1  SaveFormat=Structure With Time  SampleTime=-1
  To Workspace2 : ToWorkspace  VariableName=samp_2  SaveFormat=Structure With Time  SampleTime=-1
  To Workspace3 : ToWorkspace  VariableName=samp_3  SaveFormat=Structure With Time  SampleTime=-1
  To Workspace4 : ToWorkspace  VariableName=samp_4  SaveFormat=Structure With Time  SampleTime=-1
  To Workspace5 : ToWorkspace  VariableName=samp_5  SaveFormat=Structure With Time  SampleTime=-1
  To Workspace6 : ToWorkspace  VariableName=samp_6  SaveFormat=Structure With Time  SampleTime=-1
  To Workspace7 : ToWorkspace  VariableName=samp_7  SaveFormat=Structure With Time  SampleTime=-1
  wires:
  Real-Imag to Complex6/1 -> Spectrum Analyzer2/2, To Workspace5/1
  im_5/1 -> Real-Imag to Complex6/2, Scope/11
  re_5/1 -> Real-Imag to Complex6/1, Scope/12
  Real-Imag to Complex5/1 -> Spectrum Analyzer2/1, To Workspace4/1
  Real-Imag to Complex3/1 -> Spectrum Analyzer5/2, To Workspace1/1
  Real-Imag to Complex1/1 -> Spectrum Analyzer5/1, To Workspace/1
  Real-Imag to Complex7/1 -> Spectrum Analyzer3/1, To Workspace6/1
  im_7/1 -> Real-Imag to Complex8/2, Scope/15
  re_3/1 -> Real-Imag to Complex4/1, Scope/8
  re_7/1 -> Real-Imag to Complex8/1, Scope/16
  Real-Imag to Complex4/1 -> Spectrum Analyzer4/2, To Workspace3/1
  re_2/1 -> Real-Imag to Complex2/1, Scope/6
  re_4/1 -> Real-Imag to Complex5/1, Scope/10
  im_2/1 -> Real-Imag to Complex2/2, Scope/5
  re_0/1 -> Real-Imag to Complex1/1, Scope/2
  re_6/1 -> Real-Imag to Complex7/1, Scope/14
  im_6/1 -> Real-Imag to Complex7/2, Scope/13
  Real-Imag to Complex8/1 -> Spectrum Analyzer3/2, To Workspace7/1
  im_3/1 -> Real-Imag to Complex4/2, Scope/7
  Real-Imag to Complex2/1 -> Spectrum Analyzer4/1, To Workspace2/1
  im_4/1 -> Real-Imag to Complex5/2, Scope/9
  im_1/1 -> Real-Imag to Complex3/2, Scope/3
  re_1/1 -> Real-Imag to Complex3/1, Scope/4
  im_0/1 -> Real-Imag to Complex1/2, Scope/1

== system HLS_VMC_testing/Testing Rig/Subsystem1 ==
  Chirp : dspsrcs4/Chirp  sweep=Quadratic  mode=Unidirectional  f0=100  f1=2500  t1=0.5  Tsweep=0.5  phase=0  Ts=1/10000  spf=1  datatype=double  OutputFrames=off
  Chirp1 : dspsrcs4/Chirp  sweep=Quadratic  mode=Unidirectional  f0=100  f1=2500  t1=0.5  Tsweep=0.5  phase=pi  Ts=1/10000  spf=1  datatype=double  OutputFrames=off
  Data Type Conversion : hlsBasic/Data Type Conversion  OutDataType=data type expression  TypeExp='x_sfix64_En63'  Signedness=Signed  WordLength=16  FractionalLength=0  RoundingMode=Truncation to minus infinity  OverflowMode=Wrap around
  Data Type Conversion1 : hlsBasic/Data Type Conversion  OutDataType=data type expression  TypeExp='x_sfix64_En63'  Signedness=Signed  WordLength=16  FractionalLength=0  RoundingMode=Truncation to minus infinity  OverflowMode=Wrap around
  Gateway In : hdlBasic/Gateway In  Commented=through  gui_display_data_type=Fixed-point  arith_type=Signed (2's comp)  n_bits=32  bin_pt=31  preci_type=Single  exp_width=8  frac_width=24  rows=1  columns=1  quantization="Round  (unbiased: +/- Inf)"  overflow=Saturate  period=1/10000  UseAsADC=off  ADCChannel='1'  interface=None  automatic_assignment=on  address_offset=hex2dec('00')  intf_name=''  intf_description=''  default_value=0  timing_constraint=None  locs_specified=off  LOCs={}  io_standard={}  inherit_from_input=off  hdl_port=on  XmcBlockStatus=1  maskContainerNames=group4  block_type=gatewayin  block_config=sysgen:gateway_in_config  block_width_w=590  block_height_w=620  block_width=640  block_height=850
  Gateway In1 : hdlBasic/Gateway In  Commented=through  gui_display_data_type=Fixed-point  arith_type=Signed (2's comp)  n_bits=32  bin_pt=31  preci_type=Single  exp_width=8  frac_width=24  rows=1  columns=1  quantization="Round  (unbiased: +/- Inf)"  overflow=Saturate  period=1/10000  UseAsADC=off  ADCChannel='1'  interface=None  automatic_assignment=on  address_offset=hex2dec('00')  intf_name=''  intf_description=''  default_value=0  timing_constraint=None  locs_specified=off  LOCs={}  io_standard={}  inherit_from_input=off  hdl_port=on  XmcBlockStatus=1  maskContainerNames=group4  block_type=gatewayin  block_config=sysgen:gateway_in_config  block_width_w=590  block_height_w=620  block_width=640  block_height=850
  Real-Imag to Complex : hlsBasic/Real-Imag to Complex  Input=Real and imag  ConstantPart=0
  Scope1 : Scope
      settings: ActiveDisplayYMinimum=-0.49999999999999989  ActiveDisplayYMaximum=4.5
  Scope2 : Scope
      settings: ActiveDisplayYMinimum=-1.2499961853027344  ActiveDisplayYMaximum=1.2499656677246094  DataLoggingVariableName=ScopeData2
  Sine Wave : dspsrcs4/Sine Wave  Amplitude=1  Frequency=1000  Phase=0  SampleMode=Discrete  OutComplex=Real  CompMethod=Trigonometric fcn  TableSize=Speed  SampleTime=1/fs  SamplesPerFrame=1  ResetState=Restart at time zero  OutputFrames=off  dataType=double  wordLen=16  udDataType=sfix(16)  fracBitsMode=Best precision  numFracBits=15  OutDataTypeStr=double  LastOutDataTypeStr=double
  Sine Wave1 : dspsrcs4/Sine Wave  Amplitude=1  Frequency=1000  Phase=pi  SampleMode=Discrete  OutComplex=Real  CompMethod=Trigonometric fcn  TableSize=Speed  SampleTime=1/fs  SamplesPerFrame=1  ResetState=Restart at time zero  OutputFrames=off  dataType=double  wordLen=16  udDataType=sfix(16)  fracBitsMode=Best precision  numFracBits=15  OutDataTypeStr=double  LastOutDataTypeStr=double
  Spectrum Analyzer1 : SpectrumAnalyzer  WindowPosition=[674.000000,55.000000,800.000000,500.000000,]  ScopeFrameLocation=window  ViewType=Spectrum and spectrogram  WindowInvariantSamplesPerUpdate=on  YLimits=[-82.4589 1.756]  ColorLimits=[-82.4589 1.756]
  Step : Step  After=4  SampleTime=1/fs  ZeroCross=off
  Step1 : Step  After=4  SampleTime=1/fs  ZeroCross=off
  Out1 : Outport
  wires:
  Data Type Conversion1/1 -> Real-Imag to Complex/1
  Gateway In/1 -> Scope2/1, Data Type Conversion1/1
  Gateway In1/1 -> Spectrum Analyzer1/1, Data Type Conversion/1
  Data Type Conversion/1 -> Real-Imag to Complex/2
  Real-Imag to Complex/1 -> Out1/1, Scope1/1
  Sine Wave1/1 -> Gateway In/1
  Sine Wave/1 -> Gateway In1/1
